simulink model "part2"  (R2023b)
settings: Solver=VariableStepAuto  StartTime=0.0  StopTime=1  RelTol=1e-3
libraries: dspstat3 x3, dspmathops x3, dspfdesign x2, dspsrcs4 x1, simulink x1, spsTriangleGeneratorLib x1
settings Model: Creator=henry  LastModifiedBy=henry

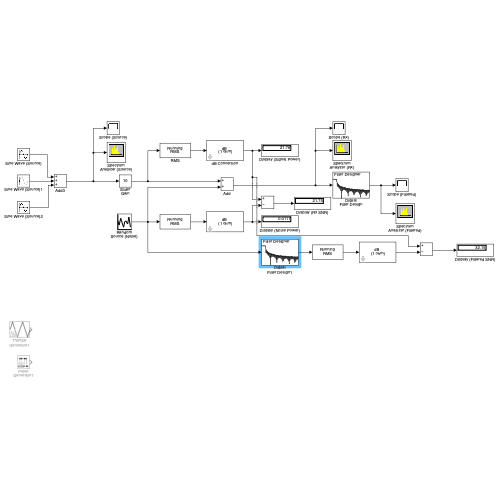
[thumbnail: Simulink's stored preview of the top-level diagram]
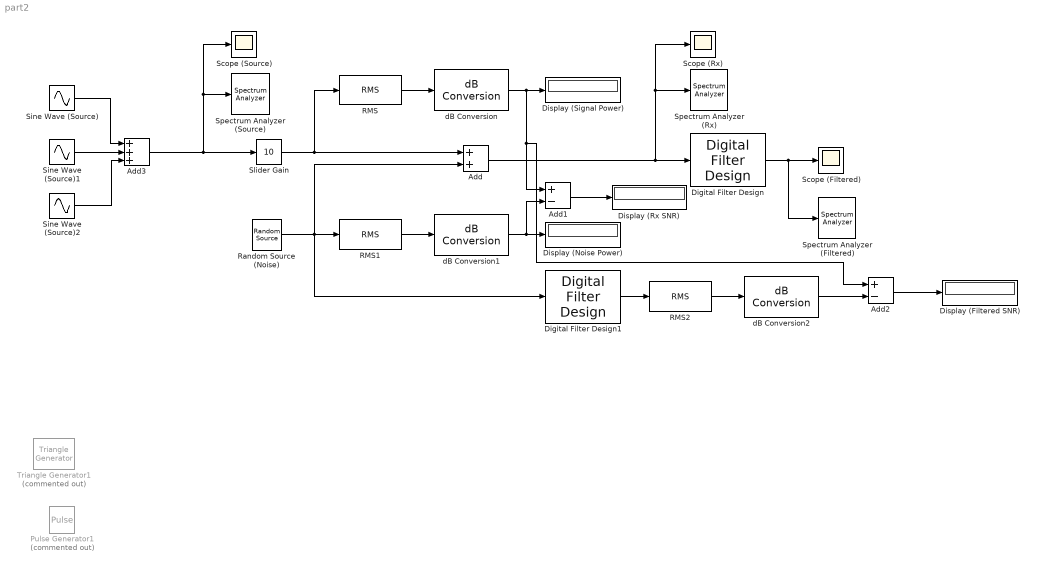
== system part2 ==
  Add : Sum
  Add1 : Sum  Inputs=+-
  Add2 : Sum  Inputs=+-
  Add3 : Sum  Inputs=+++
  Digital Filter Design : dspfdesign/Digital Filter Design  mwdsp_browser_bugfix_var=off
  Digital Filter Design1 : dspfdesign/Digital Filter Design  mwdsp_browser_bugfix_var=off
  Display (Filtered SNR) : Display
  Display (Noise Power) : Display
  Display (Rx SNR) : Display
  Display (Signal Power) : Display
  Pulse Generator1 : DiscretePulseGenerator  Commented=on  Period=100  PulseWidth=80  SampleTime=1e-6
  RMS : dspstat3/RMS  run=on  directionMode=Each column  dimension=1  InputProcessing=Columns as channels (frame based)  reset_popup=None
  RMS1 : dspstat3/RMS  run=on  directionMode=Each column  dimension=1  InputProcessing=Columns as channels (frame based)  reset_popup=None
  RMS2 : dspstat3/RMS  run=on  directionMode=Each column  dimension=1  InputProcessing=Columns as channels (frame based)  reset_popup=None
  Random Source (Noise) : dspsrcs4/Random Source  SrcType=Gaussian  NormMethod=Ziggurat  CltLength=12  MinVal=0  MaxVal=1  MeanVal=0  VarVal=1  RepMode=Not repeatable  rawSeed=1  IsInherit=off  SampMode=Discrete  SampTime=1e-6  SampFrame=1  DataType=Double  OutComplex=Real  OutputFrames=off
  Scope (Filtered) : Scope
  Scope (Rx) : Scope
  Scope (Source) : Scope
  Sine Wave (Source) : Sin  SineType=Sample based  Samples=50  SampleTime=1e-6
  Sine Wave (Source)1 : Sin  SineType=Sample based  Samples=100  SampleTime=1e-6
  Sine Wave (Source)2 : Sin  SineType=Sample based  Samples=200  SampleTime=1e-6
  Slider Gain : simulink/Math Operations/Slider Gain  gain=10  low=0  high=20
  Spectrum Analyzer (Filtered) : SpectrumAnalyzer  WindowPosition=[340.000000,151.000000,800.000000,500.000000,]  ScopeFrameLocation=window  YLimits=[-78.45603409,53.21310415]
  Spectrum Analyzer (Rx) : SpectrumAnalyzer  WindowPosition=[320.000000,200.000000,800.000000,500.000000,]  ScopeFrameLocation=window  YLimits=[-10.2862539,50.01935319]
  Spectrum Analyzer (Source) : SpectrumAnalyzer  WindowPosition=[320.000000,201.000000,800.000000,500.000000,]  ScopeFrameLocation=window  YLimits=[-249.18885578,54.33142388]
  Triangle Generator1 : spsTriangleGeneratorLib/Triangle Generator  Commented=on  Freq=1e4  Phase=90  Ts=1e-6
  dB Conversion : dspmathops/dB Conversion  dBtype=dB  intype=Amplitude  R=1  fuzz=off
      settings: LibrarySourceBlock=commutil2/dB Conversion
  dB Conversion1 : dspmathops/dB Conversion  dBtype=dB  intype=Amplitude  R=1  fuzz=off
      settings: LibrarySourceBlock=commutil2/dB Conversion
  dB Conversion2 : dspmathops/dB Conversion  dBtype=dB  intype=Amplitude  R=1  fuzz=off
      settings: LibrarySourceBlock=commutil2/dB Conversion
  wires:
  Add3/1 -> Spectrum Analyzer (Source)/1, Scope (Source)/1, Slider Gain/1
  Slider Gain/1 -> RMS/1, Add/1
  RMS/1 -> dB Conversion/1
  Random Source (Noise)/1 -> Digital Filter Design1/1, RMS1/1, Add/2
  dB Conversion/1 -> Add2/1, Add1/1, Display (Signal Power)/1
  RMS1/1 -> dB Conversion1/1
  dB Conversion1/1 -> Add1/2, Display (Noise Power)/1
  Add1/1 -> Display (Rx SNR)/1
  Add/1 -> Scope (Rx)/1, Spectrum Analyzer (Rx)/1, Digital Filter Design/1
  Digital Filter Design/1 -> Spectrum Analyzer (Filtered)/1, Scope (Filtered)/1
  RMS2/1 -> dB Conversion2/1
  Digital Filter Design1/1 -> RMS2/1
  dB Conversion2/1 -> Add2/2
  Add2/1 -> Display (Filtered SNR)/1
  Sine Wave (Source)1/1 -> Add3/2
  Sine Wave (Source)/1 -> Add3/1
  Sine Wave (Source)2/1 -> Add3/3
